simulink model "testeCCFaseC"  (R2015a)
settings: Solver=FixedStepDiscrete  StartTime=0.0  StopTime=4.5  RelTol=1e-3
PreLoadFcn:
  | Ts=20e-6;
undefined symbols (not defined in the file or in its folder): driveGuiManager, gcbh, sps_rtmsupport
libraries: powerlib x19, powerlib_meascontrol x17, simulink_extras x3, spsDrivesOutputSelector x1
(part 1 of 2)
Description:
  | Copyright 2008-2015 The MathWorks, Inc.
settings Model: CovSFcnEnable=off  ExtModeAutoUpdateStatusClock=off  Creator=MathWorks  LastModifiedBy=range
settings DataIOCC: SignalLoggingSaveFormat=ModelDataLogs  SignalLoggingName=sigsOut
settings OptimizationCC: ExpressionDepthLimit=2147483647  InitFltsAndDblsToZero=on
settings DebuggingCC: UnderspecifiedInitializationDetection=Classic  MergeDetectMultiDrivingBlocksExec=none  CheckExecutionContextPreStartOutputMsg=on  CheckExecutionContextRuntimeOutputMsg=on  SignalResolutionControl=TryResolveAllWithWarning  MultiTaskDSMMsg=warning  MultiTaskCondExecSysMsg=none  FcnCallInpInsideContextMsg=UseLocalSettings  StateNameClashWarn=warning
settings HardwareCC: TargetLongLongMode=on  TargetIntDivRoundTo=Zero  TargetEndianess=LittleEndian  TargetHWDeviceType=MATLAB Host  ProdEqTarget=off
settings GRTTargetCC: CombineOutputUpdateFcns=off  GRTInterface=on

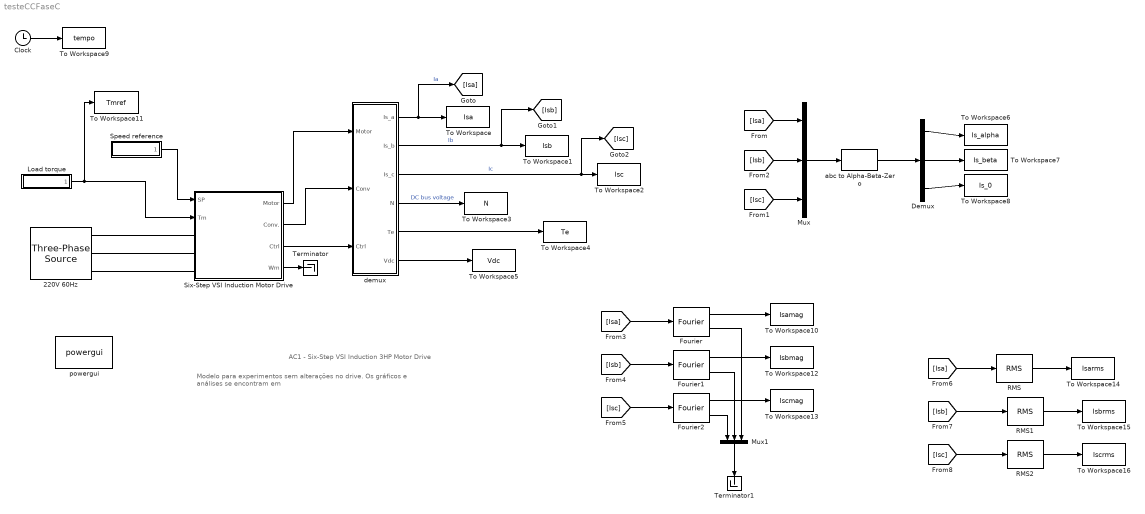
== system testeCCFaseC ==
  note: Modelo para experimentos sem alterações no drive.
      | Os gráficos e análises se encontram em
  note: AC1 - Six-Step VSI Induction 3HP Motor Drive
  220V 60Hz : powerlib/Electrical Sources/Three-Phase Source  Voltage=220  PhaseAngle=0  Frequency=60  InternalConnection=Yg  SpecifyImpedance=off  Resistance=0.1  Inductance=0.1e-3  ShortCircuitLevel=0  BaseVoltage=0  XRratio=0  BusType=swing  Pref=0  Qref=0  Qmin=-inf  Qmax=inf
  Clock : Clock
  Demux : Demux  Outputs=3
  Fourier : powerlib_meascontrol/Measurements/Fourier  Freq=60  n=1  InInit=[0, 0]  Ts=Ts
  Fourier1 : powerlib_meascontrol/Measurements/Fourier  Freq=60  n=1  InInit=[0, 0]  Ts=Ts
  Fourier2 : powerlib_meascontrol/Measurements/Fourier  Freq=60  n=1  InInit=[0, 0]  Ts=Ts
  Load torque : Subsystem
  Mux : Mux  Inputs=3
  Mux1 : Mux  Inputs=3
  RMS : powerlib_meascontrol/Measurements/RMS  TrueRMS=on  Freq=60  RMSInit=120  Ts=Ts
  RMS1 : powerlib_meascontrol/Measurements/RMS  TrueRMS=on  Freq=60  RMSInit=120  Ts=Ts
  RMS2 : powerlib_meascontrol/Measurements/RMS  TrueRMS=on  Freq=60  RMSInit=120  Ts=Ts
  Six-Step VSI Induction Motor Drive : Subsystem  LoadFcn=sps_rtmsupport('LoadFcn',gcbh); driveGuiManager('Load',get_param(gcb,'driveType'), gcbh);  StartFcn=sps_rtmsupport('StartFcn',gcbh);  StopFcn=|  mask(Six-Step VSI Induction Motor Drive){showMaskWarnings=on, AverageValue=off, MechanicalLoad=Torque Tm, driveType=AC1, outputBusMode=Multiple output buses}
      | sps_rtmsupport('StopFcn',gcbh);                                  
      | driveGuiManager('ReactivateGui',get_param(gcb,'driveType'),gcbh);
      mask prompts: showMaskWarnings "Show mask synchronization warnings"; AverageValue "Average value model"; MechanicalLoad "Mechanical input:"; driveType "Drive type:"; outputBusMode "Output bus mode:"
      mask init:
      | block=gcb;
      | [X1,X1m,X2,X2m,X3,X4,Y1,Y1m,Y2,Y2m,Y3,Y4,color1,color2,INp,OUTp,Ts,machineType] = spsDrivesMaskInit(block,driveType,AverageValue);
      | spsDrivesOutputSelectorCbak(block);
      settings: CopyFcn=sps_rtmsupport('CopyFcn',gcbh);  DeleteFcn="sps_rtmsupport('DeleteFcn',gcbh); driveGuiManager('Delete',get_param(gcb,'driveType')  ,gcbh)"  UndoDeleteFcn=sps_rtmsupport('UndoDeleteFcn',gcbh);  ModelCloseFcn=sps_rtmsupport('ModelCloseFcn',gcbh);  PreSaveFcn=sps_rtmsupport('PreSaveFcn',gcbh);  PostSaveFcn=sps_rtmsupport('PostSaveFcn',gcbh);  NameChangeFcn=sps_rtmsupport('NameChangeFcn',gcbh);  PreCopyFcn=sps_rtmsupport('PreCopyFcn',gcbh);  CloseFcn="sps_rtmsupport('CloseFcn',gcbh); driveGuiManager('Delete',get_param(gcb,'driveType')  ,gcbh);"  PreDeleteFcn=sps_rtmsupport('PreDeleteFcn',gcbh);  ParentCloseFcn="driveGuiManager('Hide',get_param(gcb,'driveType')  ,gcbh)"
      settings: OpenFcn=|
      | sps_rtmsupport('parametereditingmodes',gcbh, [1 2 3 4 5]); if (power_openblockproxy ('secondary'))
      | driveGuiManager('Create',get_param(gcb,'driveType')  ,gcbh)
      | end;
      mask Help: helpview(psbhelp)
      mask TypeOptions MechanicalLoad: Torque Tm | Speed w | Mechanical rotational port
      mask TypeOptions driveType: AC1
      mask TypeOptions outputBusMode: Multiple output buses | Single output bus
      mask Display:
      | patch([X1 X1m],[Y1 Y1m],color1);
      | patch(X3,Y3,color2);
      | plot([X1 X1m X2 X2m X3 X4],[Y1 Y1m Y2 Y2m Y3 Y4]);
      | text(0.5,0.3,'AC1','HorizontalAlignment','center')
      | HaveSPSMec = (strcmp(MechanicalLoad,'Torque Tm') || strcmp(MechanicalLoad,'Speed w'));
      | if (HaveSPSMec==1 && strcmp(outputBusMode,'Multiple output buses'))
      |     port_label('input',2,INp)
      |     port_label('output',4,OUTp)
      | end
      | if (HaveSPSMec==1 && strcmp(outputBusMode,'Single output bus'))
      |     port_label('input',2,INp)
      |     port_label('output',2,OUTp)
      | end
  Speed reference : Subsystem
  Terminator : Terminator
  Terminator1 : Terminator
  To Workspace : ToWorkspace  VariableName=Isa  SampleTime=-1
  To Workspace1 : ToWorkspace  VariableName=Isb  SampleTime=-1
  To Workspace10 : ToWorkspace  VariableName=Isamag  SampleTime=-1
  To Workspace11 : ToWorkspace  VariableName=Tmref  SampleTime=-1
  To Workspace12 : ToWorkspace  VariableName=Isbmag  SampleTime=-1
  To Workspace13 : ToWorkspace  VariableName=Iscmag  SampleTime=-1
  To Workspace14 : ToWorkspace  VariableName=Isarms  SampleTime=-1
  To Workspace15 : ToWorkspace  VariableName=Isbrms  SampleTime=-1
  To Workspace16 : ToWorkspace  VariableName=Iscrms  SampleTime=-1
  To Workspace2 : ToWorkspace  VariableName=Isc  SampleTime=-1
  To Workspace3 : ToWorkspace  VariableName=N  SampleTime=-1
  To Workspace4 : ToWorkspace  VariableName=Te  SampleTime=-1
  To Workspace5 : ToWorkspace  VariableName=Vdc  SampleTime=-1
  To Workspace6 : ToWorkspace  VariableName=Is_alpha  SampleTime=-1
  To Workspace7 : ToWorkspace  VariableName=Is_beta  SampleTime=-1
  To Workspace8 : ToWorkspace  VariableName=Is_0  SampleTime=-1
  To Workspace9 : ToWorkspace  VariableName=tempo  SampleTime=-1
  abc to Alpha-Beta-Zero : powerlib_meascontrol/Transformations/abc to Alpha-Beta-Zero
  demux : Subsystem
  powergui : powerlib/powergui  Priority=2  SimulationMode=Discrete  SolverType=Tustin/Backward Euler (TBE)  SampleTime=Ts  frequency=60  SPID=off  DisableSnubberDevices=off  DisableRonSwitches=off  DisableVfSwitches=off  SwTol=0  DisplayEquations=off  Interpol=off  methode=off  Ts=0  FunctionMessages=off  echomessages=off  HookPort=off  EnableUseOfTLC=off  x0status=blocks  frequencyindice=60  Pbase=100e6  ErrMax=1e-4  Iterations=50  UnitsV=kV  UnitsW=MW  buscounter=0  RestoreLinks=warning  ResistiveCurrentMeasurement=off  Frange=[0:2:500]  Ylog=off  Xlog=on  ShowGrid=off  save=off  variable=ZData  structure=0  ZoomFFT=on  StartTime=0.0  cycles=1  DisplayStyle=1  fundamental=60  FreqAxis=off  MaxFrequency=1000  frequencyindicesteady=1  RmsSteady=1  display=off
  wires:
  Speed reference/1(" ") -> Six-Step VSI Induction Motor Drive/1(SP)
  Load torque/1(" ") -> To Workspace11/1, Six-Step VSI Induction Motor Drive/2(Tm)
  Six-Step VSI Induction Motor Drive/1(Motor) -> demux/1(Motor)
  Six-Step VSI Induction Motor Drive/2(Conv.) -> demux/2(Conv)
  Six-Step VSI Induction Motor Drive/3(Ctrl) -> demux/3(Ctrl)
  Six-Step VSI Induction Motor Drive/4(Wm) -> Terminator/1
  demux/1(Is_a) -> To Workspace/1, [Isa]  "Ia"
  demux/2(Is_b) -> To Workspace1/1, [Isb]  "Ib"
  demux/3(Is_c) -> To Workspace2/1, [Isc]  "Ic"
  demux/4(N) -> To Workspace3/1  "DC bus voltage"
  demux/5(Te) -> To Workspace4/1
  demux/6(Vdc) -> To Workspace5/1
  Mux/1 -> abc to Alpha-Beta-Zero/1
  [Isa] -> Mux/1
  [Isb] -> Mux/2
  [Isc] -> Mux/3
  abc to Alpha-Beta-Zero/1 -> Demux/1
  Demux/1 -> To Workspace6/1
  Demux/2 -> To Workspace7/1
  Demux/3 -> To Workspace8/1
  Clock/1 -> To Workspace9/1
  [Isa] -> Fourier/1
  [Isb] -> Fourier1/1
  [Isc] -> Fourier2/1
  Fourier/1 -> To Workspace10/1
  Fourier1/1 -> To Workspace12/1
  Fourier2/1 -> To Workspace13/1
  Mux1/1 -> Terminator1/1
  Fourier2/2 -> Mux1/1
  Fourier1/2 -> Mux1/2
  Fourier/2 -> Mux1/3
  [Isa] -> RMS/1
  RMS/1 -> To Workspace14/1
  [Isb] -> RMS1/1
  RMS1/1 -> To Workspace15/1
  RMS2/1 -> To Workspace16/1
  [Isc] -> RMS2/1
  connections:
  220V 60Hz/RConn1 -- Six-Step VSI Induction Motor Drive/LConn1
  220V 60Hz/RConn2 -- Six-Step VSI Induction Motor Drive/LConn2
  220V 60Hz/RConn3 -- Six-Step VSI Induction Motor Drive/LConn3

== system testeCCFaseC/Load torque ==
  Stair Generator : powerlib_meascontrol/Pulse & Signal Generators/Stair Generator  t=[0. 1.]  e=[0. 7.7]  Ts=Ts
  " " : Outport
  wires:
  Stair Generator/1 -> " "/1

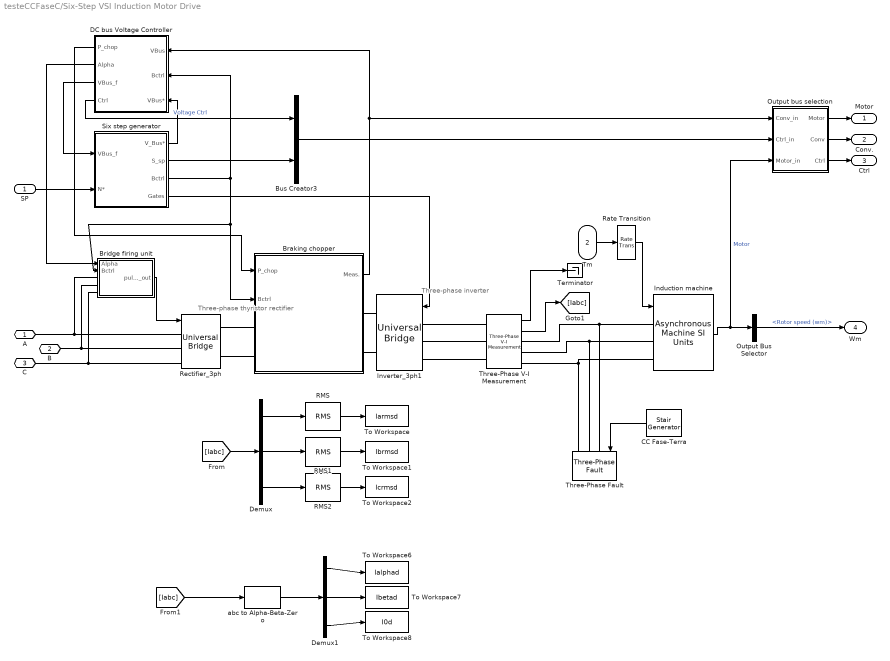
== system testeCCFaseC/Six-Step VSI Induction Motor Drive ==
  note: Three-phase
      | thyristor rectifier
  note: Three-phase
      | inverter
  SP : Inport
  Tm : Inport  Port=2
  Braking chopper : Subsystem  mask(DC bus){ind_bus=1e-3, cap_bus=4000e-6, Br=8, freq_chop=4000}
      mask prompts: ind_bus "DC bus filter - inductance (H)"; cap_bus "DC bus filter - capacitance (F)"; Br "Braking resistance (ohms)"; freq_chop "Chopper frequency (Hz)"
      mask help: This block contains a passive LC filter. The capacitor is used to provide energy to the motor. The braking chopper reduces the bus voltage during breaking mode.
      mask init:
      | [X1,X1m,X2,X2m,X3,X4,Y1,Y1m,Y2,Y2m,Y3,Y4,color1,color2]=spsdrivelogo;
      mask Display:
      | patch([X1 X1m],[Y1 Y1m],color1);
      | patch(X3,Y3,color2);
      | plot([X1 X1m X2 X2m X3 X4],[Y1 Y1m Y2 Y2m Y3 Y4]);
  Bridge firing unit : Subsystem  mask(Bridge firing unit){net_f=60}
      mask prompts: net_f "Network frequency (Hz)"
      mask help: This block implements a six pulse firing unit with notch filter. The phase sequence must stay ABC.
  Bus Creator3 : BusCreator  Inputs=2
  CC Fase-Terra : powerlib_meascontrol/Pulse & Signal Generators/Stair Generator  t=[2]  e=[1]  Ts=Ts
  DC bus Voltage Controller : Subsystem  mask(DC bus voltage controller){ki=0.1, kp=0.01, fc=30, Ts=Ts}
      mask prompts: ki "Integral gain"; kp "Proportional gain"; fc "DC bus voltage measurement - low-pass filter cutoff frequency (Hz)"; Ts "Simulation time step (s)"
      mask help: The PI controller of the DC bus voltage.
      mask init:
      | [X1,X1m,X2,X2m,X3,X4,Y1,Y1m,Y2,Y2m,Y3,Y4,color1,color2]=spsdrivelogo;
      mask Display:
      | patch([X1 X1m],[Y1 Y1m],color1);
      | patch(X3,Y3,color2);
      | plot([X1 X1m X2 X2m X3 X4],[Y1 Y1m Y2 Y2m Y3 Y4]);
  Demux : Demux  Outputs=3
  Demux1 : Demux  Outputs=3
  Induction machine : powerlib/Machines/Asynchronous Machine SI Units  RotorType=Squirrel-cage  PresetModel=No  MechanicalLoad=Torque Tm  ShowDetailedParameters=on  ReferenceFrame=Stationary  Units=SI  MeasurementBus=off  NominalParameters=[2238,220,60]  Stator=[0.435,0.002]  Rotor=[0.816,0.002]  Cage1=[ 0.022 0.226/377]  Cage2=[ 0.022 0.226/377]  Lm=69.31e-3  Mechanical=[0.089,0.005,2]  PolePairs=2  InitialConditions=[1,0,0,0,0,0,0,0]  SimulateSaturation=off  Saturation=[0 0;0 0]  LoadFlowParameters=0  TsPowergui=0  TsBlock=-1  IterativeModel=Trapezoidal non iterative  Pmec=0
  Inverter_3ph1 : powerlib/Power Electronics/Universal Bridge  Arms=3  SnubberResistance=1e3  SnubberCapacitance=20e-9  Device=IGBT / Diodes  Ron=1e-3  Lon=0  ForwardVoltages=[1.7,1.7]  ForwardVoltage=0  GTOparameters=[10e-6,20e-6]  IGBTparameters=[1e-6,2e-6]  Measurements=All voltages and currents  Measurements_2=None  converterType=Inverter
  Output Bus Selector : BusSelector  OutputSignals=Mechanical.Rotor speed (wm)
  Output bus selection : Subsystem  BlockChoice=Multiple output buses
      settings: AttributesFormatString=%<BlockChoice>  TemplateBlock=spsDrivesOutputSelector/Output bus selection  MemberBlocks=Multiple output buses,Single output bus
  RMS : powerlib_meascontrol/Measurements/RMS  TrueRMS=on  Freq=60  RMSInit=120  Ts=Ts
  RMS1 : powerlib_meascontrol/Measurements/RMS  TrueRMS=on  Freq=60  RMSInit=120  Ts=Ts
  RMS2 : powerlib_meascontrol/Measurements/RMS  TrueRMS=on  Freq=60  RMSInit=120  Ts=Ts
  Rate Transition : RateTransition  OutPortSampleTime=Ts
  Rectifier_3ph : powerlib/Power Electronics/Universal Bridge  Arms=3  SnubberResistance=5e3  SnubberCapacitance=100e-9  Device=Thyristors  Ron=1e-3  Lon=0  ForwardVoltages="[  0  0  ]"  ForwardVoltage=1.3  GTOparameters=[ 10e-6 , 20e-6 ]  IGBTparameters=[ 1e-6 , 2e-6 ]  Measurements=None  Measurements_2=None  converterType=Rectifier
  Six step generator : Subsystem  mask(Six step generator){p=2, pos_dv=20, neg_dv=20, decel_ramp=-2000, accel_ramp=2000, minof=0, maxof=120, minbv=30, maxbv=280, vbhr=5, zc_time=0.5}
      mask prompts: p "Motor pairs of poles"; pos_dv "DC bus positive deviation (V)"; neg_dv "DC bus negative deviation (V)"; decel_ramp "Deceleration ramp (rpm/sec)"; accel_ramp "Acceleration ramp (rpm/sec)"; minof "Minimum output frequency (Hz)"; maxof "Maximum output frequency (Hz)"; minbv "Minimum bus voltage (V)"; maxbv "Maximum bus voltage (V)"; vbhr "Volts/Hertz ratio (V/Hz)"; zc_time "Zero speed crossing time (s)"
      mask help: This block implements a six step generator. A braking and motoring logic can toggle between the braking chopper and the thyristor bridge.
      mask init:
      | [X1,X1m,X2,X2m,X3,X4,Y1,Y1m,Y2,Y2m,Y3,Y4,color1,color2]=spsdrivelogo;
      mask Display:
      | patch([X1 X1m],[Y1 Y1m],color1);
      | patch(X3,Y3,color2);
      | plot([X1 X1m X2 X2m X3 X4],[Y1 Y1m Y2 Y2m Y3 Y4]);
  Terminator : Terminator
  Three-Phase V-I Measurement : powerlib/Measurements/Three-Phase V-I Measurement  VoltageMeasurement=phase-to-ground  SetLabelV=off  LabelV=Vabc  Vpu=off  VpuLL=off  CurrentMeasurement=yes  SetLabelI=off  LabelI=Iabc  Ipu=off  Pbase=100e6  Vbase=500e3  OutputType=Complex  PhasorSimulation=off  PSBequivalent=0
  Three-Phase Fault : powerlib/Elements/Three-Phase Fault  InitialStates=0  FaultA=off  FaultB=off  FaultC=on  GroundFault=on  SwitchTimes="[1/60  5/60]"  External=on  SwitchStatus=NaN  FaultResistance=0.001  GroundResistance=0.01  SnubberResistance=1e6  SnubberCapacitance=inf  Measurements=None
  To Workspace : ToWorkspace  VariableName=Iarmsd  SampleTime=-1
  To Workspace1 : ToWorkspace  VariableName=Ibrmsd  SampleTime=-1
  To Workspace2 : ToWorkspace  VariableName=Icrmsd  SampleTime=-1
  To Workspace6 : ToWorkspace  VariableName=Ialphad  SampleTime=-1
  To Workspace7 : ToWorkspace  VariableName=Ibetad  SampleTime=-1
  To Workspace8 : ToWorkspace  VariableName=I0d  SampleTime=-1
  abc to Alpha-Beta-Zero : powerlib_meascontrol/Transformations/abc to Alpha-Beta-Zero
  A : PMIOPort  Port=1  Side=Left
  B : PMIOPort  Port=2  Side=Left
  C : PMIOPort  Port=3  Side=Left
  Motor : Outport
  Conv. : Outport  Port=2
  Ctrl : Outport  Port=3
  Wm : Outport  Port=4
  wires:
  Output bus selection/3(Ctrl) -> Ctrl/1
  Output bus selection/2(Conv) -> Conv./1
  Output bus selection/1(Motor) -> Motor/1
  Six step generator/4(Gates) -> Inverter_3ph1/1
  Six step generator/3("Bctrl ") -> DC bus Voltage Controller/2(Bctrl), Bridge firing unit/2("Bctrl "), Braking chopper/2("Bctrl ")
  Six step generator/2(S_sp) -> Bus Creator3/2
  DC bus Voltage Controller/1(P_chop) -> Braking chopper/1(P_chop)
  Bridge firing unit/1(pulse_out) -> Rectifier_3ph/1
  DC bus Voltage Controller/2(Alpha) -> Bridge firing unit/1(Alpha)
  Induction machine/1 -> Output Bus Selector/1, Output bus selection/3(Motor_in)  "Motor"
  Bus Creator3/1 -> Output bus selection/2(Ctrl_in)
  DC bus Voltage Controller/3(VBus_f) -> Six step generator/1(VBus_f)
  SP/1 -> Six step generator/2(N*)
  Six step generator/1(V_Bus*) -> DC bus Voltage Controller/3(VBus*)
  Braking chopper/1(Meas.) -> DC bus Voltage Controller/1(VBus), Output bus selection/1(Conv_in)
  DC bus Voltage Controller/4(Ctrl) -> Bus Creator3/1  "Voltage Ctrl"
  Output Bus Selector/1 -> Wm/1  "<Rotor speed (wm)>"
  Tm/1 -> Rate Transition/1
  Rate Transition/1 -> Induction machine/1
  CC Fase-Terra/1 -> Three-Phase Fault/1
  Three-Phase V-I Measurement/2 -> [Iabc]
  Three-Phase V-I Measurement/1 -> Terminator/1
  [Iabc] -> Demux/1
  Demux/1 -> RMS/1
  RMS/1 -> To Workspace/1
  Demux/2 -> RMS1/1
  RMS1/1 -> To Workspace1/1
  Demux/3 -> RMS2/1
  RMS2/1 -> To Workspace2/1
  abc to Alpha-Beta-Zero/1 -> Demux1/1
  Demux1/1 -> To Workspace6/1
  Demux1/2 -> To Workspace7/1
  Demux1/3 -> To Workspace8/1
  [Iabc] -> abc to Alpha-Beta-Zero/1
  connections:
  C/RConn1 -- Bridge firing unit/LConn3 -- Rectifier_3ph/LConn3
  A/RConn1 -- Bridge firing unit/LConn1 -- Rectifier_3ph/LConn1
  Inverter_3ph1/RConn2 -- Braking chopper/RConn2
  Inverter_3ph1/RConn1 -- Braking chopper/RConn1
  Rectifier_3ph/LConn2 -- Bridge firing unit/LConn2 -- B/RConn1
  Rectifier_3ph/RConn2 -- Braking chopper/LConn2
  Rectifier_3ph/RConn1 -- Braking chopper/LConn1
  Induction machine/LConn2 -- Three-Phase V-I Measurement/RConn2 -- Three-Phase Fault/LConn2
  Three-Phase Fault/LConn3 -- Three-Phase V-I Measurement/RConn3 -- Induction machine/LConn3
  Three-Phase Fault/LConn1 -- Three-Phase V-I Measurement/RConn1 -- Induction machine/LConn1
  Three-Phase V-I Measurement/LConn1 -- Inverter_3ph1/LConn1
  Three-Phase V-I Measurement/LConn3 -- Inverter_3ph1/LConn3
  Three-Phase V-I Measurement/LConn2 -- Inverter_3ph1/LConn2

== system testeCCFaseC/Speed reference ==
  Stair Generator : powerlib_meascontrol/Pulse & Signal Generators/Stair Generator  t=[0]  e=[1800]  Ts=Ts
  " " : Outport
  wires:
  Stair Generator/1 -> " "/1

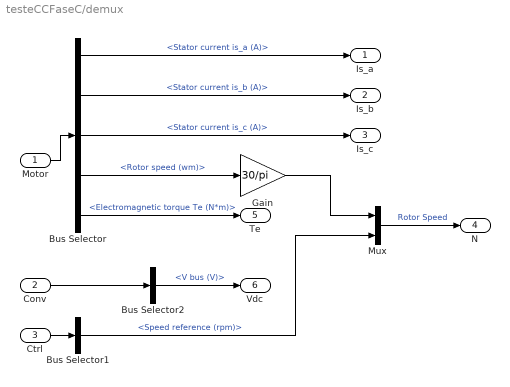
== system testeCCFaseC/demux ==
  Motor : Inport
  Conv : Inport  Port=2
  Ctrl : Inport  Port=3
  Bus Selector : BusSelector  OutputSignals=Stator measurements.Stator current is_a (A),Stator measurements.Stator current is_b (A),Stator measurements.Stator current is_c (A),Mechanical.Rotor speed (wm),Mechanical.Electromagnetic torque Te (N*m)
  Bus Selector1 : BusSelector  OutputSignals=Speed reference (rpm)
  Bus Selector2 : BusSelector  OutputSignals=V bus (V)
  Gain : Gain  Gain=30/pi  SaturateOnIntegerOverflow=on  OutDataTypeStr=Inherit: Same as input  ParamDataTypeStr=Inherit: Same as input
  Mux : Mux  Inputs=2
  Is_a : Outport
  Is_b : Outport  Port=2
  Is_c : Outport  Port=3
  N : Outport  Port=4
  Te : Outport  Port=5
  Vdc : Outport  Port=6
  wires:
  Bus Selector/4 -> Gain/1  "<Rotor speed (wm)>"
  Gain/1 -> Mux/1
  Bus Selector1/1 -> Mux/2  "<Speed reference (rpm)>"
  Bus Selector/1 -> Is_a/1  "<Stator current is_a (A)>"
  Motor/1 -> Bus Selector/1
  Conv/1 -> Bus Selector2/1
  Ctrl/1 -> Bus Selector1/1
  Bus Selector/3 -> Is_c/1  "<Stator current is_c (A)>"
  Bus Selector/2 -> Is_b/1  "<Stator current is_b (A)>"
  Mux/1 -> N/1  "Rotor Speed"
  Bus Selector/5 -> Te/1  "<Electromagnetic torque Te (N*m)>"
  Bus Selector2/1 -> Vdc/1  "<V bus (V)>"

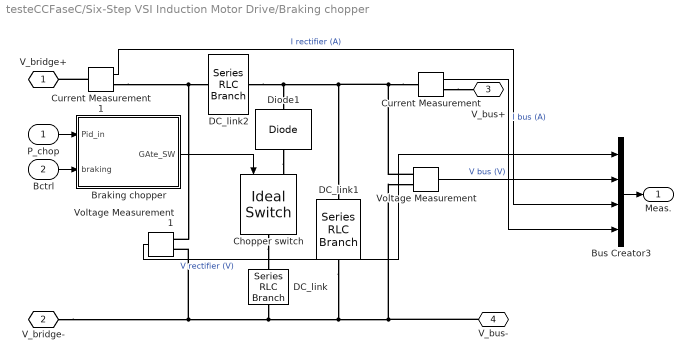
== system testeCCFaseC/Six-Step VSI Induction Motor Drive/Braking chopper ==
  P_chop : Inport
  "Bctrl " : Inport  Port=2
  Braking chopper : Subsystem
  Bus Creator3 : BusCreator
  Chopper switch : powerlib/Power Electronics/Ideal Switch  Ron=1e-3  Lon=0  IC=0  Rs=10e3  Cs=inf  Measurements=off
      settings: AttributesFormatString=\n
  Current Measurement : powerlib/Measurements/Current Measurement  PhasorSimulation=off  OutputType=Complex  PSBequivalent=0
  Current Measurement1 : powerlib/Measurements/Current Measurement  PhasorSimulation=off  OutputType=Complex  PSBequivalent=0
  DC_link : powerlib/Elements/Series RLC Branch  LConnTagsString=__new0  RConnTagsString=__new0  BranchType=R  Resistance=Br  Inductance=[]  SetiL0=off  InitialCurrent=0  Capacitance=[]  Setx0=off  InitialVoltage=0  Measurements=None
  DC_link1 : powerlib/Elements/Series RLC Branch  LConnTagsString=__new0  RConnTagsString=__new0  BranchType=C  Resistance=[]  Inductance=[]  SetiL0=off  InitialCurrent=0  Capacitance=cap_bus  Setx0=off  InitialVoltage=0  Measurements=None
  DC_link2 : powerlib/Elements/Series RLC Branch  LConnTagsString=__new0  RConnTagsString=__new0  BranchType=L  Resistance=[]  Inductance=ind_bus  SetiL0=off  InitialCurrent=0  Capacitance=[]  Setx0=off  InitialVoltage=0  Measurements=None
  Diode1 : powerlib/Power Electronics/Diode  Ron=1e-3  Lon=0  Vf=0.8  IC=0  UseSnubber=off  Rs=10e3  Cs=inf  Measurements=off
  Voltage Measurement : powerlib/Measurements/Voltage Measurement  Tag=PoWeRsYsTeMmEaSuReMeNt  PhasorSimulation=off  OutputType=Magnitude  PSBequivalent=0
  Voltage Measurement1 : powerlib/Measurements/Voltage Measurement  Tag=PoWeRsYsTeMmEaSuReMeNt  PhasorSimulation=off  OutputType=Magnitude  PSBequivalent=0
  V_bridge+ : PMIOPort  Port=1  Side=Left
  V_bridge- : PMIOPort  Port=2  Side=Left
  V_bus+ : PMIOPort  Port=3  Side=Right
  V_bus- : PMIOPort  Port=4  Side=Right
  Meas. : Outport
  wires:
  Current Measurement/1 -> Bus Creator3/4  "I bus (A)"
  Current Measurement1/1 -> Bus Creator3/3  "I rectifier (A)"
  Voltage Measurement1/1 -> Bus Creator3/1  "V rectifier (V)"
  Voltage Measurement/1 -> Bus Creator3/2  "V bus (V)"
  Bus Creator3/1 -> Meas./1
  Braking chopper/1(GAte_SW) -> Chopper switch/1
  "Bctrl "/1 -> Braking chopper/2(braking)
  P_chop/1 -> Braking chopper/1(Pid_in)
  connections:
  Current Measurement1/LConn1 -- V_bridge+/RConn1
  Voltage Measurement1/LConn1 -- DC_link2/LConn1 -- Current Measurement1/RConn1
  Current Measurement/RConn1 -- V_bus+/RConn1
  Chopper switch/RConn1 -- DC_link/LConn1
  Diode1/RConn1 -- Chopper switch/LConn1
  Current Measurement/LConn1 -- DC_link1/LConn1 -- Diode1/LConn1 -- DC_link2/RConn1 -- Voltage Measurement/LConn1
  Voltage Measurement1/LConn2 -- V_bus-/RConn1 -- Voltage Measurement/LConn2 -- DC_link1/RConn1 -- DC_link/RConn1 -- V_bridge-/RConn1

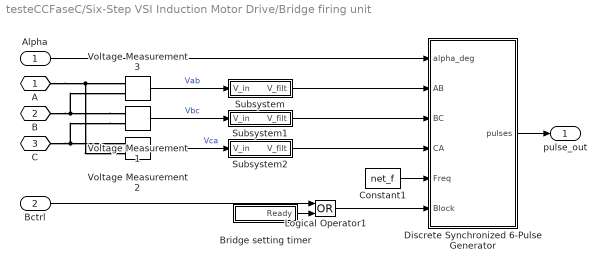
== system testeCCFaseC/Six-Step VSI Induction Motor Drive/Bridge firing unit ==
  Alpha : Inport
  "Bctrl " : Inport  Port=2
  Bridge setting timer : Subsystem
  Constant1 : Constant  Value=net_f
  Discrete Synchronized 6-Pulse Generator : Subsystem  DialogController=POWERSYS.PowerSysDialog  mask(Discrete Synchronized 6-pulse generator){pwidth=10, Double_Pulse=on, Ts=Ts}
      mask prompts: pwidth "Pulse width (degrees) :"; Double_Pulse "Double pulsing"; Ts "Time step (s) :"
      mask help:
      | Use this block to fire the 6 thyristors of a 6-pulse converter.
      |
      | The output is a vector of 6 pulses (0-1) individually synchronized on the 6 commutation voltages. Pulses are generated alpha degrees after the increasing zero-crossings of the commutation voltages.
      |
      | Input 1 is  the alpha firing signal (degrees).
      | Inputs 2, 3 and 4 are the synchronization voltages AB BC CA which should be in phase with the 3 phase-phase voltages at the converter terminals.
      | Input 5: Frequency of the synchronization voltages (use a constant or the Freq PLL output)
      | Input 6 allows  blocking of the pulses when the applied signal is non zero.
      |
      | When the 'Douple pulsing' option is checked, two pulses are sent to each thyristor: a 1st pulse when the aplha angle is reached, then a 2nd pulse 60 degrees later, when the next thyristor is fired.
      mask init:
      | power_initmask();
      mask Help: This block is part of a subset of blocks in the Extras library that does not have documentation associated with it, other than the block mask description.
      mask Display: plot(0,0,100,100,[80 62 62 47 47 30],[40 40 60 60 40 40]-5)
  Logical Operator1 : Logic  Operator=OR
  Subsystem : Subsystem
  Subsystem1 : Subsystem
  Subsystem2 : Subsystem
  Voltage Measurement1 : powerlib/Measurements/Voltage Measurement  Tag=PoWeRsYsTeMmEaSuReMeNt  PhasorSimulation=off  OutputType=Complex  PSBequivalent=0
  Voltage Measurement2 : powerlib/Measurements/Voltage Measurement  Tag=PoWeRsYsTeMmEaSuReMeNt  PhasorSimulation=off  OutputType=Complex  PSBequivalent=0
  Voltage Measurement3 : powerlib/Measurements/Voltage Measurement  Tag=PoWeRsYsTeMmEaSuReMeNt  PhasorSimulation=off  OutputType=Complex  PSBequivalent=0
  A : PMIOPort  Port=1  Side=Left
  B : PMIOPort  Port=2  Side=Left
  C : PMIOPort  Port=3  Side=Left
  pulse_out : Outport
  wires:
  Voltage Measurement2/1 -> Subsystem2/1(V_in)  "Vca"
  Voltage Measurement1/1 -> Subsystem1/1(V_in)  "Vbc"
  Voltage Measurement3/1 -> Subsystem/1(V_in)  "Vab"
  "Bctrl "/1 -> Logical Operator1/1
  Bridge setting timer/1(Ready) -> Logical Operator1/2
  Logical Operator1/1 -> Discrete Synchronized 6-Pulse Generator/6(Block)
  Constant1/1 -> Discrete Synchronized 6-Pulse Generator/5(Freq)
  Alpha/1 -> Discrete Synchronized 6-Pulse Generator/1(alpha_deg)
  Subsystem1/1(V_filt) -> Discrete Synchronized 6-Pulse Generator/3(BC)
  Subsystem2/1(V_filt) -> Discrete Synchronized 6-Pulse Generator/4(CA)
  Subsystem/1(V_filt) -> Discrete Synchronized 6-Pulse Generator/2(AB)
  Discrete Synchronized 6-Pulse Generator/1(pulses) -> pulse_out/1
  connections:
  Voltage Measurement2/LConn2 -- A/RConn1 -- Voltage Measurement3/LConn1
  Voltage Measurement1/LConn2 -- Voltage Measurement2/LConn1 -- C/RConn1
  Voltage Measurement1/LConn1 -- Voltage Measurement3/LConn2 -- B/RConn1

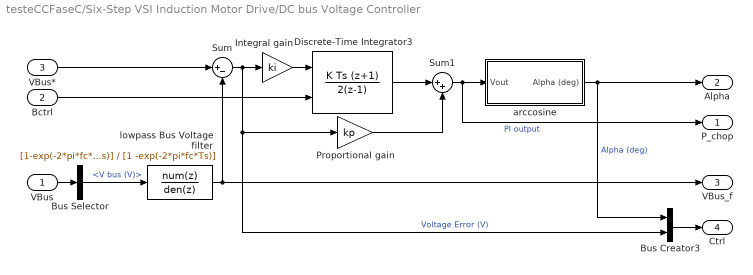
== system testeCCFaseC/Six-Step VSI Induction Motor Drive/DC bus Voltage Controller ==
  VBus : Inport
  Bctrl : Inport  Port=2
  VBus* : Inport  Port=3
  Bus Creator3 : BusCreator  Inputs=2
  Bus Selector : BusSelector  OutputSignals=V bus (V)
  Discrete-Time Integrator3 : DiscreteIntegrator  IntegratorMethod=Integration: Trapezoidal  ExternalReset=level  SampleTime=Ts  LimitOutput=on  UpperSaturationLimit=1  LowerSaturationLimit=-1
  Integral gain : Gain  Gain=ki  SaturateOnIntegerOverflow=on  OutDataTypeStr=Inherit: Same as input  ParamDataTypeStr=Inherit: Same as input
  Proportional gain : Gain  Gain=kp  SaturateOnIntegerOverflow=on  OutDataTypeStr=Inherit: Same as input  ParamDataTypeStr=Inherit: Same as input
  Sum : Sum  Inputs=|+-  SaturateOnIntegerOverflow=on  InputSameDT=on  OutDataTypeStr=Inherit: Same as first input
  Sum1 : Sum  Inputs=|++  SaturateOnIntegerOverflow=on  InputSameDT=on  OutDataTypeStr=Inherit: Same as first input
  arccosine : Subsystem
  lowpass Bus Voltage filter : DiscreteTransferFcn  Numerator=[1-exp(-2*pi*fc*Ts)]  Denominator=[1 -exp(-2*pi*fc*Ts)]  SampleTime=Ts
  P_chop : Outport
  Alpha : Outport  Port=2
  VBus_f : Outport  Port=3
  Ctrl : Outport  Port=4
  wires:
  VBus*/1 -> Sum/1
  Sum/1 -> Integral gain/1, Proportional gain/1, Bus Creator3/2  "Voltage Error (V)"
  Sum1/1 -> arccosine/1(Vout), P_chop/1  "PI output"
  Proportional gain/1 -> Sum1/2
  Discrete-Time Integrator3/1 -> Sum1/1
  Integral gain/1 -> Discrete-Time Integrator3/1
  arccosine/1(Alpha (deg)) -> Alpha/1, Bus Creator3/1  "Alpha (deg)"
  Bus Creator3/1 -> Ctrl/1
  VBus/1 -> Bus Selector/1
  Bus Selector/1 -> lowpass Bus Voltage filter/1  "<V bus (V)>"
  Bctrl/1 -> Discrete-Time Integrator3/2
  lowpass Bus Voltage filter/1 -> Sum/2, VBus_f/1

== system testeCCFaseC/Six-Step VSI Induction Motor Drive/Output bus selection ==
  Conv_in : Inport
  Ctrl_in : Inport  Port=2
  Motor_in : Inport  Port=3
  Multiple output buses : spsDrivesOutputSelector/Multiple output buses
  Motor : Outport
  Conv : Outport  Port=2
  Ctrl : Outport  Port=3
  wires:
  Conv_in/1 -> Multiple output buses/1
  Ctrl_in/1 -> Multiple output buses/2
  Motor_in/1 -> Multiple output buses/3
  Multiple output buses/1 -> Motor/1
  Multiple output buses/2 -> Conv/1
  Multiple output buses/3 -> Ctrl/1

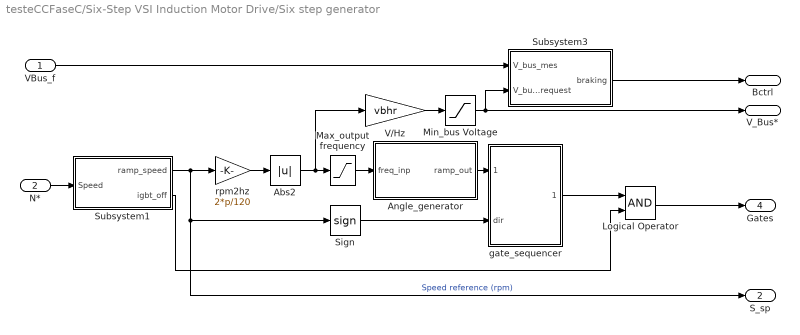
== system testeCCFaseC/Six-Step VSI Induction Motor Drive/Six step generator ==
  VBus_f : Inport
  N* : Inport  Port=2
  Abs2 : Abs  SaturateOnIntegerOverflow=on
  Angle_generator : Subsystem
  Logical Operator : Logic
  Max_output frequency : Saturate  UpperLimit=maxof  LowerLimit=minof
  Min_bus Voltage : Saturate  UpperLimit=maxbv  LowerLimit=minbv
  Sign : Signum
  Subsystem1 : Subsystem
  Subsystem3 : Subsystem
  V/Hz : Gain  Gain=vbhr  SaturateOnIntegerOverflow=on  OutDataTypeStr=Inherit: Same as input  ParamDataTypeStr=Inherit: Same as input
  gate_sequencer : Subsystem
  rpm2hz : Gain  Gain=2*p/120  SaturateOnIntegerOverflow=on  OutDataTypeStr=Inherit: Same as input  ParamDataTypeStr=Inherit: Same as input
  V_Bus* : Outport
  S_sp : Outport  Port=2
  "Bctrl " : Outport  Port=3
  Gates : Outport  Port=4
  wires:
  Subsystem1/2(igbt_off) -> Logical Operator/2
  Logical Operator/1 -> Gates/1
  gate_sequencer/1(gate_logic) -> Logical Operator/1
  Subsystem3/1(braking) -> "Bctrl "/1
  VBus_f/1 -> Subsystem3/1(V_bus_mes)
  Subsystem1/1(ramp_speed) -> S_sp/1, Sign/1, rpm2hz/1  "Speed reference (rpm)"
  Min_bus Voltage/1 -> V_Bus*/1, Subsystem3/2(V_bus_request)
  V/Hz/1 -> Min_bus Voltage/1
  Sign/1 -> gate_sequencer/2(dir)
  Angle_generator/1(ramp_out) -> gate_sequencer/1(ramp_inp)
  Max_output frequency/1 -> Angle_generator/1(freq_inp)
  Abs2/1 -> V/Hz/1, Max_output frequency/1
  N*/1 -> Subsystem1/1(Speed)
  rpm2hz/1 -> Abs2/1

== system testeCCFaseC/Six-Step VSI Induction Motor Drive/Braking chopper/Braking chopper ==
  Pid_in : Inport
  braking : Inport  Port=2
  Data Type Conversion : DataTypeConversion  SaturateOnIntegerOverflow=on  RndMeth=Zero
  Data Type Conversion1 : DataTypeConversion  SaturateOnIntegerOverflow=on  RndMeth=Zero
  Gain : Gain  Gain=-1  SaturateOnIntegerOverflow=on  OutDataTypeStr=Inherit: Same as input  ParamDataTypeStr=Inherit: Same as input
  Product : Product  SaturateOnIntegerOverflow=on  InputSameDT=on  OutDataTypeStr=Inherit: Same as first input
  Relational Operator : RelationalOperator  InputSameDT=on
  Unit Delay : UnitDelay  SampleTime=Ts
  ramp_generator : Subsystem
  GAte_SW : Outport
  wires:
  ramp_generator/1(ramp_out) -> Relational Operator/2
  braking/1 -> Data Type Conversion1/1
  Product/1 -> GAte_SW/1
  Relational Operator/1 -> Data Type Conversion/1
  Unit Delay/1 -> Relational Operator/1
  Gain/1 -> Unit Delay/1
  Pid_in/1 -> Gain/1
  Data Type Conversion/1 -> Product/1
  Data Type Conversion1/1 -> Product/2

== system testeCCFaseC/Six-Step VSI Induction Motor Drive/Bridge firing unit/Bridge setting timer ==
  Clock : Clock
  Constant2 : Constant  Value=5e-3
  Relational Operator : RelationalOperator  Operator=<=  InputSameDT=on
  Ready : Outport
  wires:
  Relational Operator/1 -> Ready/1
  Constant2/1 -> Relational Operator/2
  Clock/1 -> Relational Operator/1

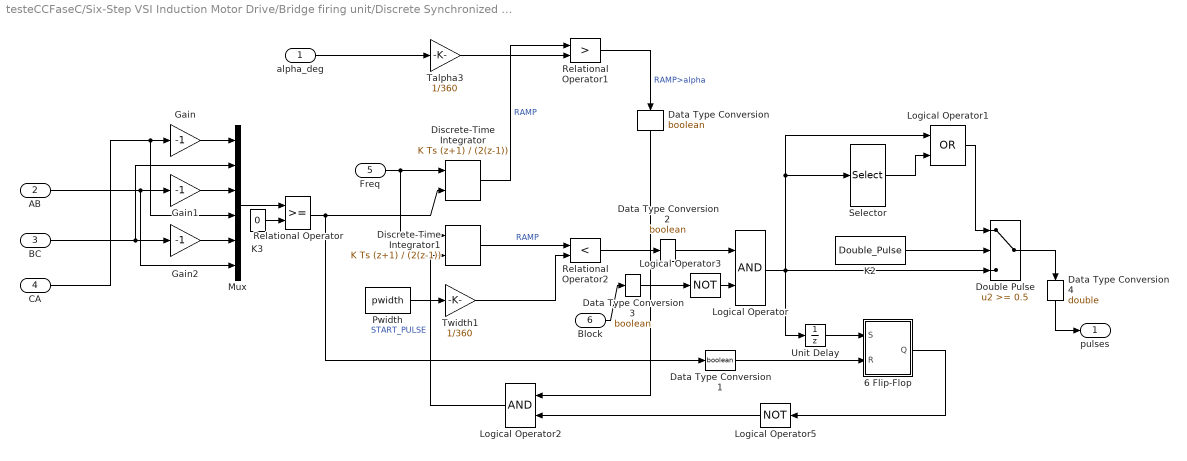
== system testeCCFaseC/Six-Step VSI Induction Motor Drive/Bridge firing unit/Discrete Synchronized 6-Pulse Generator ==
  alpha_deg : Inport
  AB : Inport  Port=2
  BC : Inport  Port=3
  CA : Inport  Port=4
  Freq : Inport  Port=5
  Block : Inport  Port=6
  6 Flip-Flop : Subsystem
  Data Type Conversion{,1..3} (4 alike) : DataTypeConversion  OutDataTypeStr=boolean  SaturateOnIntegerOverflow=on  RndMeth=Zero
  Data Type Conversion4 : DataTypeConversion  OutDataTypeStr=double  SaturateOnIntegerOverflow=on  RndMeth=Zero
  Discrete-Time Integrator : DiscreteIntegrator  IntegratorMethod=Integration: Trapezoidal  ExternalReset=rising  SampleTime=Ts
  Discrete-Time Integrator1 : DiscreteIntegrator  IntegratorMethod=Integration: Trapezoidal  ExternalReset=rising  SampleTime=Ts
  Double Pulse : Switch  Threshold=0.5  InputSameDT=on
  Gain : Gain  Gain=-1  SaturateOnIntegerOverflow=on  OutDataTypeStr=Inherit: Same as input  ParamDataTypeStr=Inherit: Same as input
  Gain1 : Gain  Gain=-1  SaturateOnIntegerOverflow=on  OutDataTypeStr=Inherit: Same as input  ParamDataTypeStr=Inherit: Same as input
  Gain2 : Gain  Gain=-1  SaturateOnIntegerOverflow=on  OutDataTypeStr=Inherit: Same as input  ParamDataTypeStr=Inherit: Same as input
  K2 : Constant  Value=Double_Pulse
  K3 : Constant  Value=0
  Logical Operator : Logic
  Logical Operator1 : Logic  Operator=OR
  Logical Operator2 : Logic
  Logical Operator3 : Logic  Operator=NOT  Inputs=1
  Logical Operator5 : Logic  Operator=NOT  Inputs=1
  Mux : Mux  Inputs=6
  Pwidth : Constant  Value=pwidth
  Relational Operator : RelationalOperator  InputSameDT=on
  Relational Operator1 : RelationalOperator  Operator=>  InputSameDT=on
  Relational Operator2 : RelationalOperator  Operator=<  InputSameDT=on
  Selector : Selector  InputPortWidth=6  Indices=[2 3 4 5 6 1 ]
  Talpha3 : Gain  Gain=1/360  SaturateOnIntegerOverflow=on  OutDataTypeStr=Inherit: Same as input  ParamDataTypeStr=Inherit: Same as input
  Twidth1 : Gain  Gain=1/360  SaturateOnIntegerOverflow=on  OutDataTypeStr=Inherit: Same as input  ParamDataTypeStr=Inherit: Same as input
  Unit Delay : UnitDelay  SampleTime=Ts
  pulses : Outport  InitialOutput=0
  wires:
  alpha_deg/1 -> Talpha3/1
  6 Flip-Flop/1(Q) -> Logical Operator5/1
  Freq/1 -> Discrete-Time Integrator1/1, Discrete-Time Integrator/1
  BC/1 -> Mux/2, Gain2/1
  CA/1 -> Mux/4, Gain/1
  Mux/1 -> Relational Operator/1
  Talpha3/1 -> Relational Operator1/2
  Logical Operator5/1 -> Logical Operator2/2
  Relational Operator/1 -> Discrete-Time Integrator/2, Data Type Conversion1/1
  K3/1 -> Relational Operator/2
  Gain2/1 -> Mux/5
  Gain1/1 -> Mux/3
  Gain/1 -> Mux/1
  Discrete-Time Integrator/1 -> Relational Operator1/1  "RAMP"
  Discrete-Time Integrator1/1 -> Relational Operator2/1  "RAMP"
  Twidth1/1 -> Relational Operator2/2
  Pwidth/1 -> Twidth1/1
  Logical Operator1/1 -> Double Pulse/1
  Selector/1 -> Logical Operator1/2
  Logical Operator/1 -> Logical Operator1/1, Selector/1, Double Pulse/3, Unit Delay/1
  K2/1 -> Double Pulse/2
  Unit Delay/1 -> 6 Flip-Flop/1(S)
  Logical Operator3/1 -> Logical Operator/2
  AB/1 -> Gain1/1, Mux/6
  Logical Operator2/1 -> Discrete-Time Integrator1/2  "START_PULSE"
  Relational Operator1/1 -> Data Type Conversion/1  "RAMP>alpha"
  Data Type Conversion/1 -> Logical Operator2/1
  Data Type Conversion1/1 -> 6 Flip-Flop/2(R)
  Relational Operator2/1 -> Data Type Conversion2/1
  Data Type Conversion2/1 -> Logical Operator/1
  Block/1 -> Data Type Conversion3/1
  Data Type Conversion3/1 -> Logical Operator3/1
  Double Pulse/1 -> Data Type Conversion4/1
  Data Type Conversion4/1 -> pulses/1

== system testeCCFaseC/Six-Step VSI Induction Motor Drive/Bridge firing unit/Subsystem ==
  V_in : Inport
  Second-Order Filter : powerlib_meascontrol/Filters/Second-Order Filter  FilterType=Bandstop (Notch)  Fo=net_f  Zeta=0.1  Ts=Ts  Initialize=on  Vac_Init=[310*sin(30*pi/180) 30 net_f]  Vdc_Init=0  PlotResponse=off  FreqRange=[0, 500, 1]
  Sum1 : Sum  Inputs=|-+  SaturateOnIntegerOverflow=on  InputSameDT=on  OutDataTypeStr=Inherit: Same as first input
  V_filt : Outport
  wires:
  Sum1/1 -> V_filt/1
  Second-Order Filter/1 -> Sum1/1
  V_in/1 -> Sum1/2, Second-Order Filter/1

== system testeCCFaseC/Six-Step VSI Induction Motor Drive/Bridge firing unit/Subsystem1 ==
  V_in : Inport
  Second-Order Filter : powerlib_meascontrol/Filters/Second-Order Filter  FilterType=Bandstop (Notch)  Fo=net_f  Zeta=0.1  Ts=Ts  Initialize=on  Vac_Init=[310*sin(pi/2) -90 net_f]  Vdc_Init=0  PlotResponse=off  FreqRange=[0, 500, 1]
  Sum1 : Sum  Inputs=|-+  SaturateOnIntegerOverflow=on  InputSameDT=on  OutDataTypeStr=Inherit: Same as first input
  V_filt : Outport
  wires:
  V_in/1 -> Sum1/2, Second-Order Filter/1
  Second-Order Filter/1 -> Sum1/1
  Sum1/1 -> V_filt/1

== system testeCCFaseC/Six-Step VSI Induction Motor Drive/Bridge firing unit/Subsystem2 ==
  V_in : Inport
  Second-Order Filter : powerlib_meascontrol/Filters/Second-Order Filter  FilterType=Bandstop (Notch)  Fo=net_f  Zeta=0.1  Ts=Ts  Initialize=on  Vac_Init=[310*sin(150*pi/180) 150 net_f]  Vdc_Init=0  PlotResponse=off  FreqRange=[0, 500, 1]
  Sum1 : Sum  Inputs=|-+  SaturateOnIntegerOverflow=on  InputSameDT=on  OutDataTypeStr=Inherit: Same as first input
  V_filt : Outport
  wires:
  Sum1/1 -> V_filt/1
  Second-Order Filter/1 -> Sum1/1
  V_in/1 -> Sum1/2, Second-Order Filter/1

== system testeCCFaseC/Six-Step VSI Induction Motor Drive/DC bus Voltage Controller/arccosine ==
  Vout : Inport
  0 <Vout<1 : Fcn  Expr=acos(u(1))-pi/3
  0.5<Vout<1 : Fcn  Expr=acos(u(1))
  Alpha4 : Constant  Value=0.5
  Rad2Deg : Gain  Gain=180/pi  SaturateOnIntegerOverflow=on  OutDataTypeStr=Inherit: Same as input  ParamDataTypeStr=Inherit: Same as input
  Relational Operator : RelationalOperator  OutDataTypeStr=boolean
  Saturation1 : Saturate  UpperLimit=1  LowerLimit=-1
  Saturation2 : Saturate  UpperLimit=inf  LowerLimit=0.0001
  Saturation3 : Saturate  UpperLimit=1  LowerLimit=-1
  Switch : Switch  Threshold=0.5
  u(1)-1 : Fcn  Expr=u(1)-1
  Alpha (deg) : Outport
  wires:
  Rad2Deg/1 -> Saturation2/1
  Alpha4/1 -> Relational Operator/2
  Relational Operator/1 -> Switch/2
  0.5<Vout<1/1 -> Switch/1
  0 <Vout<1/1 -> Switch/3
  u(1)-1/1 -> Saturation1/1
  Saturation1/1 -> 0 <Vout<1/1
  Switch/1 -> Rad2Deg/1
  Saturation3/1 -> 0.5<Vout<1/1
  Vout/1 -> Relational Operator/1, u(1)-1/1, Saturation3/1
  Saturation2/1 -> Alpha (deg)/1

== system testeCCFaseC/Six-Step VSI Induction Motor Drive/Six step generator/Angle_generator ==
  freq_inp : Inport
  Constant : Constant  Value=360
  Constant1 : Constant  Value=360
  Discrete-Time Integrator1 : DiscreteIntegrator  IntegratorMethod=Integration: Trapezoidal  ExternalReset=rising  SampleTime=Ts
  Product : Product  SaturateOnIntegerOverflow=on  InputSameDT=on  OutDataTypeStr=Inherit: Same as first input
  Relational Operator : RelationalOperator  InputSameDT=on
  Unit Delay : UnitDelay  SampleTime=Ts
  ramp_out : Outport
  wires:
  freq_inp/1 -> Product/2
  Product/1 -> Discrete-Time Integrator1/1
  Constant1/1 -> Product/1
  Unit Delay/1 -> Discrete-Time Integrator1/2
  Relational Operator/1 -> Unit Delay/1
  Constant/1 -> Relational Operator/2
  Discrete-Time Integrator1/1 -> ramp_out/1, Relational Operator/1

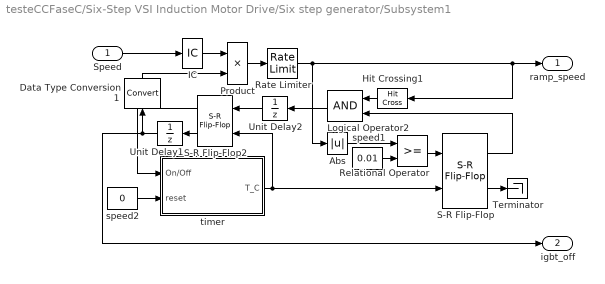
== system testeCCFaseC/Six-Step VSI Induction Motor Drive/Six step generator/Subsystem1 ==
  Speed : Inport
  Abs : Abs  SaturateOnIntegerOverflow=on
  Data Type Conversion1 : DataTypeConversion  SaturateOnIntegerOverflow=on  RndMeth=Zero
  Hit Crossing1 : HitCross
  IC : InitialCondition  Value=0
  Logical Operator2 : Logic
  Product : Product  SaturateOnIntegerOverflow=on  InputSameDT=on  OutDataTypeStr=Inherit: Same as first input
  Rate Limiter : RateLimiter  RisingSlewLimit=accel_ramp  FallingSlewLimit=decel_ramp
  Relational Operator : RelationalOperator  InputSameDT=on
  S-R Flip-Flop : simulink_extras/Flip Flops/S-R Flip-Flop  initial_condition=0
  S-R Flip-Flop2 : simulink_extras/Flip Flops/S-R Flip-Flop  initial_condition=0
  Terminator : Terminator
  Unit Delay1 : UnitDelay  SampleTime=Ts
  Unit Delay2 : UnitDelay  SampleTime=Ts
  speed1 : Constant  Value=0.01
  speed2 : Constant  Value=0
  timer : Subsystem
  ramp_speed : Outport
  igbt_off : Outport  Port=2
  wires:
  Logical Operator2/1 -> Unit Delay2/1
  S-R Flip-Flop/1 -> Logical Operator2/2
  Hit Crossing1/1 -> Logical Operator2/1
  S-R Flip-Flop/2 -> Terminator/1
  Abs/1 -> Relational Operator/1
  speed2/1 -> timer/2(reset)
  timer/1(T_C) -> S-R Flip-Flop/2, S-R Flip-Flop2/2
  Unit Delay2/1 -> S-R Flip-Flop2/1
  S-R Flip-Flop2/1 -> timer/1(On/Off)
  Unit Delay1/1 -> igbt_off/1, Data Type Conversion1/1
  Relational Operator/1 -> S-R Flip-Flop/1
  S-R Flip-Flop2/2 -> Unit Delay1/1
  IC/1 -> Product/1
  Rate Limiter/1 -> Hit Crossing1/1, ramp_speed/1, Abs/1
  Product/1 -> Rate Limiter/1
  Speed/1 -> IC/1
  speed1/1 -> Relational Operator/2
  Data Type Conversion1/1 -> Product/2

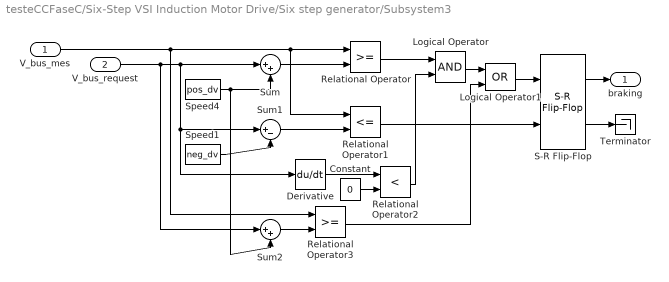
== system testeCCFaseC/Six-Step VSI Induction Motor Drive/Six step generator/Subsystem3 ==
  V_bus_mes : Inport
  V_bus_request : Inport  Port=2
  Constant : Constant  Value=0
  Derivative : Derivative
  Logical Operator : Logic
  Logical Operator1 : Logic  Operator=OR
  Relational Operator : RelationalOperator  InputSameDT=on
  Relational Operator1 : RelationalOperator  Operator=<=  InputSameDT=on
  Relational Operator2 : RelationalOperator  Operator=<  InputSameDT=on
  Relational Operator3 : RelationalOperator  InputSameDT=on
  S-R Flip-Flop : simulink_extras/Flip Flops/S-R Flip-Flop  initial_condition=0
  Speed1 : Constant  Value=neg_dv
  Speed4 : Constant  Value=pos_dv
  Sum : Sum  Inputs=|++  SaturateOnIntegerOverflow=on  InputSameDT=on  OutDataTypeStr=Inherit: Same as first input
  Sum1 : Sum  Inputs=|+-  SaturateOnIntegerOverflow=on  InputSameDT=on  OutDataTypeStr=Inherit: Same as first input
  Sum2 : Sum  Inputs=|++  SaturateOnIntegerOverflow=on  InputSameDT=on  OutDataTypeStr=Inherit: Same as first input
  Terminator : Terminator
  braking : Outport
  wires:
  Speed1/1 -> Sum1/2
  Relational Operator3/1 -> Logical Operator1/2
  Logical Operator1/1 -> S-R Flip-Flop/1
  S-R Flip-Flop/1 -> braking/1
  Logical Operator/1 -> Logical Operator1/1
  Relational Operator2/1 -> Logical Operator/2
  Relational Operator/1 -> Logical Operator/1
  Sum2/1 -> Relational Operator3/2
  Constant/1 -> Relational Operator2/2
  Derivative/1 -> Relational Operator2/1
  V_bus_request/1 -> Sum2/1, Derivative/1, Sum1/1, Sum/1
  V_bus_mes/1 -> Relational Operator3/1, Relational Operator1/1, Relational Operator/1
  S-R Flip-Flop/2 -> Terminator/1
  Speed4/1 -> Sum/2, Sum2/2
  Sum1/1 -> Relational Operator1/2
  Sum/1 -> Relational Operator/2
  Relational Operator1/1 -> S-R Flip-Flop/2

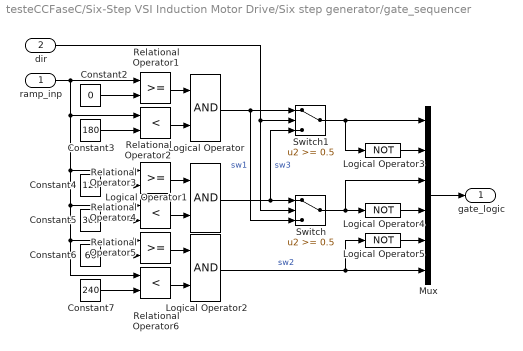
== system testeCCFaseC/Six-Step VSI Induction Motor Drive/Six step generator/gate_sequencer ==
  ramp_inp : Inport
  dir : Inport  Port=2
  Constant2 : Constant  Value=0
  Constant3 : Constant  Value=180
  Constant4 : Constant  Value=120
  Constant5 : Constant  Value=300
  Constant6 : Constant  Value=60
  Constant7 : Constant  Value=240
  Logical Operator : Logic
  Logical Operator1 : Logic
  Logical Operator2 : Logic
  Logical Operator3 : Logic  Operator=NOT
  Logical Operator4 : Logic  Operator=NOT
  Logical Operator5 : Logic  Operator=NOT
  Mux : Mux  Inputs=6
  Relational Operator1 : RelationalOperator  InputSameDT=on
  Relational Operator2 : RelationalOperator  Operator=<  InputSameDT=on
  Relational Operator3 : RelationalOperator  InputSameDT=on
  Relational Operator4 : RelationalOperator  Operator=<  InputSameDT=on
  Relational Operator5 : RelationalOperator  InputSameDT=on
  Relational Operator6 : RelationalOperator  Operator=<  InputSameDT=on
  Switch : Switch  Threshold=0.5  SaturateOnIntegerOverflow=on  InputSameDT=on
  Switch1 : Switch  Threshold=0.5  SaturateOnIntegerOverflow=on  InputSameDT=on
  gate_logic : Outport
  wires:
  ramp_inp/1 -> Relational Operator6/1, Relational Operator5/1, Relational Operator4/1, Relational Operator3/1, Relational Operator2/1, Relational Operator1/1
  Relational Operator2/1 -> Logical Operator/2
  Relational Operator1/1 -> Logical Operator/1
  Constant3/1 -> Relational Operator2/2
  Constant2/1 -> Relational Operator1/2
  Logical Operator1/1 -> Switch1/3, Switch/1  "sw3"
  dir/1 -> Switch/2, Switch1/2
  Switch/1 -> Mux/3, Logical Operator4/1
  Switch1/1 -> Logical Operator3/1, Mux/1
  Mux/1 -> gate_logic/1
  Logical Operator/1 -> Switch/3, Switch1/1  "sw1"
  Logical Operator2/1 -> Mux/6, Logical Operator5/1  "sw2"
  Logical Operator5/1 -> Mux/5
  Logical Operator4/1 -> Mux/4
  Logical Operator3/1 -> Mux/2
  Relational Operator6/1 -> Logical Operator2/2
  Relational Operator5/1 -> Logical Operator2/1
  Constant7/1 -> Relational Operator6/2
  Constant6/1 -> Relational Operator5/2
  Relational Operator4/1 -> Logical Operator1/2
  Relational Operator3/1 -> Logical Operator1/1
  Constant5/1 -> Relational Operator4/2
  Constant4/1 -> Relational Operator3/2

== system testeCCFaseC/Six-Step VSI Induction Motor Drive/Braking chopper/Braking chopper/ramp_generator ==
  Constant3 : Constant
  Discrete-Time Integrator1 : DiscreteIntegrator  ExternalReset=rising  SampleTime=Ts
  Relational Operator1 : RelationalOperator  InputSameDT=on
  Unit Delay1 : UnitDelay  SampleTime=Ts
  fc : Constant  Value=freq_chop
  ramp_out : Outport
  wires:
  Unit Delay1/1 -> Discrete-Time Integrator1/2
  Relational Operator1/1 -> Unit Delay1/1
  Constant3/1 -> Relational Operator1/2
  Discrete-Time Integrator1/1 -> ramp_out/1, Relational Operator1/1
  fc/1 -> Discrete-Time Integrator1/1

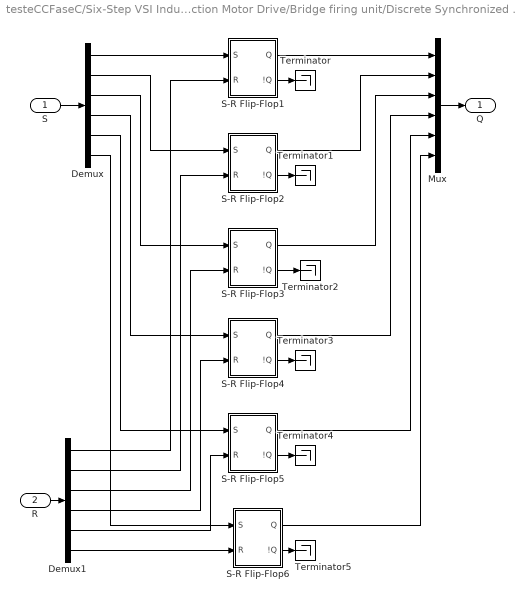
== system testeCCFaseC/Six-Step VSI Induction Motor Drive/Bridge firing unit/Discrete Synchronized 6-Pulse Generator/6 Flip-Flop ==
  S : Inport
  R : Inport  Port=2
  Demux : Demux  Outputs=6
  Demux1 : Demux  Outputs=6
  Mux : Mux  Inputs=6
  S-R Flip-Flop1 : Subsystem  mask(SRFlipFlop){initial_condition=0, Ts=Ts}
      mask prompts: initial_condition "Initial condition:"; Ts "Sample time:"
      mask help: S-R Flip Flop Block
  S-R Flip-Flop2 : Subsystem  mask(SRFlipFlop){initial_condition=0, Ts=Ts}
      mask prompts: initial_condition "Initial condition:"; Ts "Sample time:"
      mask help: S-R Flip Flop Block
  S-R Flip-Flop3 : Subsystem  mask(SRFlipFlop){initial_condition=0, Ts=Ts}
      mask prompts: initial_condition "Initial condition:"; Ts "Sample time:"
      mask help: S-R Flip Flop Block
  S-R Flip-Flop4 : Subsystem  mask(SRFlipFlop){initial_condition=0, Ts=Ts}
      mask prompts: initial_condition "Initial condition:"; Ts "Sample time:"
      mask help: S-R Flip Flop Block
  S-R Flip-Flop5 : Subsystem  mask(SRFlipFlop){initial_condition=0, Ts=Ts}
      mask prompts: initial_condition "Initial condition:"; Ts "Sample time:"
      mask help: S-R Flip Flop Block
  S-R Flip-Flop6 : Subsystem  mask(SRFlipFlop){initial_condition=0, Ts=Ts}
      mask prompts: initial_condition "Initial condition:"; Ts "Sample time:"
      mask help: S-R Flip Flop Block
  Terminator{,1..5} (6 alike) : Terminator
  Q : Outport
  wires:
  Demux1/6 -> S-R Flip-Flop6/2(R)
  Demux1/5 -> S-R Flip-Flop5/2(R)
  Demux1/4 -> S-R Flip-Flop4/2(R)
  Demux1/3 -> S-R Flip-Flop3/2(R)
  Demux1/2 -> S-R Flip-Flop2/2(R)
  Demux1/1 -> S-R Flip-Flop1/2(R)
  R/1 -> Demux1/1
  Demux/5 -> S-R Flip-Flop5/1(S)
  Demux/6 -> S-R Flip-Flop6/1(S)
  S/1 -> Demux/1
  Demux/4 -> S-R Flip-Flop4/1(S)
  Demux/3 -> S-R Flip-Flop3/1(S)
  Demux/2 -> S-R Flip-Flop2/1(S)
  Demux/1 -> S-R Flip-Flop1/1(S)
  S-R Flip-Flop1/2(!Q) -> Terminator/1
  S-R Flip-Flop6/1(Q) -> Mux/6
  Mux/1 -> Q/1
  S-R Flip-Flop5/1(Q) -> Mux/5
  S-R Flip-Flop4/1(Q) -> Mux/4
  S-R Flip-Flop3/1(Q) -> Mux/3
  S-R Flip-Flop2/1(Q) -> Mux/2
  S-R Flip-Flop1/1(Q) -> Mux/1
  S-R Flip-Flop2/2(!Q) -> Terminator1/1
  S-R Flip-Flop3/2(!Q) -> Terminator2/1
  S-R Flip-Flop4/2(!Q) -> Terminator3/1
  S-R Flip-Flop5/2(!Q) -> Terminator4/1
  S-R Flip-Flop6/2(!Q) -> Terminator5/1

== system testeCCFaseC/Six-Step VSI Induction Motor Drive/Six step generator/Subsystem1/timer ==
  On/Off : Inport
  reset : Inport  Port=2
  Data Type Conversion : DataTypeConversion  SaturateOnIntegerOverflow=on  RndMeth=Zero
  Data Type Conversion1 : DataTypeConversion  SaturateOnIntegerOverflow=on  RndMeth=Zero
  Discrete-Time Integrator : DiscreteIntegrator  IntegratorMethod=Integration: Trapezoidal  ExternalReset=level  SampleTime=Ts
  Gain : Gain  SaturateOnIntegerOverflow=on  OutDataTypeStr=Inherit: Same as input  ParamDataTypeStr=Inherit: Same as input
  Logical Operator8 : Logic  Operator=OR
  Relational Operator3 : RelationalOperator  InputSameDT=on
  Unit Delay : UnitDelay  SampleTime=Ts
  speed5 : Constant  Value=zc_time
  T_C : Outport
  wires:
  reset/1 -> Data Type Conversion/1
  Logical Operator8/1 -> Discrete-Time Integrator/2
  Unit Delay/1 -> Logical Operator8/2, T_C/1
  On/Off/1 -> Data Type Conversion1/1
  Relational Operator3/1 -> Unit Delay/1
  speed5/1 -> Relational Operator3/2
  Gain/1 -> Relational Operator3/1
  Discrete-Time Integrator/1 -> Gain/1
  Data Type Conversion/1 -> Logical Operator8/1
  Data Type Conversion1/1 -> Discrete-Time Integrator/1

== system testeCCFaseC/Six-Step VSI Induction Motor Drive/Bridge firing unit/Discrete Synchronized 6-Pulse Generator/6 Flip-Flop/S-R Flip-Flop1 ==
  S : Inport
  R : Inport  Port=2
  Demux : Demux  Outputs=2
  Logic : CombinatorialLogic  TruthTable=[0 1;0 1;1 0;0 1;1 0;0 1;1 0;1 0]
  Mux : Mux  Inputs=3
  Unit Delay : UnitDelay  InitialCondition=initial_condition  SampleTime=Ts
  Q : Outport  InitialOutput=0
  !Q : Outport  Port=2  InitialOutput=1
  wires:
  Mux/1 -> Logic/1
  Logic/1 -> Demux/1
  Demux/2 -> !Q/1
  Demux/1 -> Q/1, Unit Delay/1
  Unit Delay/1 -> Mux/1
  S/1 -> Mux/2
  R/1 -> Mux/3

== system testeCCFaseC/Six-Step VSI Induction Motor Drive/Bridge firing unit/Discrete Synchronized 6-Pulse Generator/6 Flip-Flop/S-R Flip-Flop2 ==
  S : Inport
  R : Inport  Port=2
  Demux : Demux  Outputs=2
  Logic : CombinatorialLogic  TruthTable=[0 1;0 1;1 0;0 1;1 0;0 1;1 0;1 0]
  Mux : Mux  Inputs=3
  Unit Delay : UnitDelay  InitialCondition=initial_condition  SampleTime=Ts
  Q : Outport  InitialOutput=0
  !Q : Outport  Port=2  InitialOutput=1
  wires:
  R/1 -> Mux/3
  S/1 -> Mux/2
  Unit Delay/1 -> Mux/1
  Demux/1 -> Unit Delay/1, Q/1
  Demux/2 -> !Q/1
  Logic/1 -> Demux/1
  Mux/1 -> Logic/1

== system testeCCFaseC/Six-Step VSI Induction Motor Drive/Bridge firing unit/Discrete Synchronized 6-Pulse Generator/6 Flip-Flop/S-R Flip-Flop3 ==
  S : Inport
  R : Inport  Port=2
  Demux : Demux  Outputs=2
  Logic : CombinatorialLogic  TruthTable=[0 1;0 1;1 0;0 1;1 0;0 1;1 0;1 0]
  Mux : Mux  Inputs=3
  Unit Delay : UnitDelay  InitialCondition=initial_condition  SampleTime=Ts
  Q : Outport  InitialOutput=0
  !Q : Outport  Port=2  InitialOutput=1
  wires:
  Mux/1 -> Logic/1
  Logic/1 -> Demux/1
  Demux/2 -> !Q/1
  Demux/1 -> Q/1, Unit Delay/1
  Unit Delay/1 -> Mux/1
  S/1 -> Mux/2
  R/1 -> Mux/3

== system testeCCFaseC/Six-Step VSI Induction Motor Drive/Bridge firing unit/Discrete Synchronized 6-Pulse Generator/6 Flip-Flop/S-R Flip-Flop4 ==
  S : Inport
  R : Inport  Port=2
  Demux : Demux  Outputs=2
  Logic : CombinatorialLogic  TruthTable=[0 1;0 1;1 0;0 1;1 0;0 1;1 0;1 0]
  Mux : Mux  Inputs=3
  Unit Delay : UnitDelay  InitialCondition=initial_condition  SampleTime=Ts
  Q : Outport  InitialOutput=0
  !Q : Outport  Port=2  InitialOutput=1
  wires:
  R/1 -> Mux/3
  S/1 -> Mux/2
  Unit Delay/1 -> Mux/1
  Demux/1 -> Unit Delay/1, Q/1
  Demux/2 -> !Q/1
  Logic/1 -> Demux/1
  Mux/1 -> Logic/1
